simulink model "slam_check"  (R2013b)
settings: Solver=ode3  StartTime=0.0  StopTime=3  FixedStep=0.1  RelTol=1e-3
undefined symbols (not defined in the file): DiscIntNeverNeededParam
settings Model: Creator=chida  LastModifiedBy=chida
settings DataIOCC: SignalLoggingSaveFormat=ModelDataLogs
settings DebuggingCC: MultiTaskDSMMsg=warning  MultiTaskCondExecSysMsg=none
settings RTWCC: IncludeERTFirstTime=on

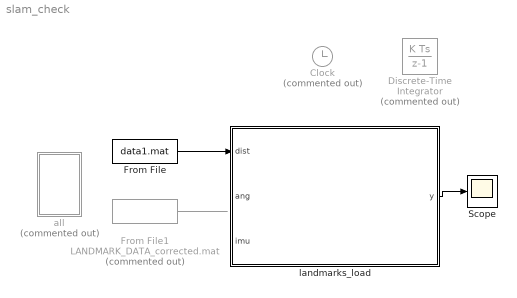
== system slam_check ==
  Clock : Clock  Commented=on
  Discrete-Time Integrator : DiscreteIntegrator  Commented=on  ICPrevOutput=DiscIntNeverNeededParam  ICPrevScaledInput=DiscIntNeverNeededParam
  From File : FromFile  FileName=data1.mat  SampleTime=0
  From File1 : FromFile  Commented=on  FileName=LANDMARK_DATA_corrected.mat  SampleTime=0
  Scope : Scope
  all : Subsystem  Commented=on
  landmarks_load : MATLAB Function  TreatAsAtomicUnit=on
  wires:
  From File/1 -> landmarks_load/1(dist)
  landmarks_load/1(y) -> Scope/1
  From File1/1 -> ?

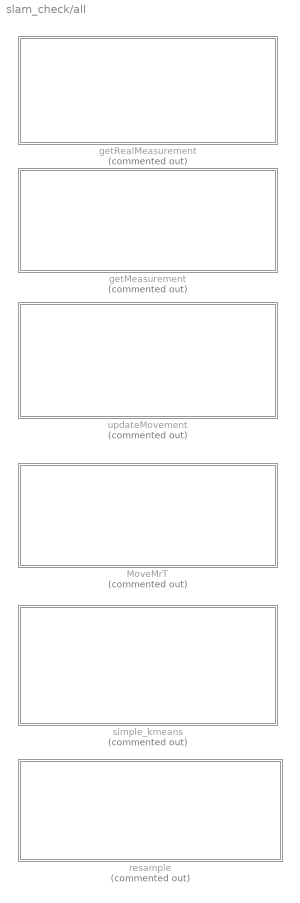
== system slam_check/all ==
  MoveMrT : MATLAB Function  Commented=on  TreatAsAtomicUnit=on
  getMeasurement : MATLAB Function  Commented=on  TreatAsAtomicUnit=on
  getRealMeasurement : MATLAB Function  Commented=on  TreatAsAtomicUnit=on
  resample : MATLAB Function  Commented=on  TreatAsAtomicUnit=on
  simple_kmeans : MATLAB Function  Commented=on  TreatAsAtomicUnit=on
  updateMovement : MATLAB Function  Commented=on  TreatAsAtomicUnit=on

== matlab function slam_check/all/getMeasurement ==
%%%%%%%%%%%%%%%%%%%%%%%%%%%%%%%%%%%%%%%%%%%%%%%%%%%%%%%%%%%%%%%%%%%%%%
%  Copyright 2010 Randolph Voorhies
%  This program is free software: you can redistribute it and/or modify
%  it under the terms of the GNU General Public License as published by
%  the Free Software Foundation, either version 3 of the License, or
%  (at your option) any later version.
%
%  This program is distributed in the hope that it will be useful,
%  but WITHOUT ANY WARRANTY; without even the implied warranty of
%  MERCHANTABILITY or FITNESS FOR A PARTICULAR PURPOSE.  See the
%  GNU General Public License for more details.
%
%  You should have received a copy of the GNU General Public License
%  along with this program.  If not, see <http://www.gnu.org/licenses/>.
%%%%%%%%%%%%%%%%%%%%%%%%%%%%%%%%%%%%%%%%%%%%%%%%%%%%%%%%%%%%%%%%%%%%%%   
% function [z, H] = getMeasurement(pos, landmark_pos, observation_variance)
function getMeasurement
%   Given a landmark position and a robot position, this method will return a
%   "measurement" z that contains the distance and the angle to the landmark.
%   Gaussian random noise is added to both based on the variances given in the
%   diagonal of the observation_variance matrix. Note that this method is used
%   both to take a "real" measurement in the simulation, as well as to assess 
%   what kind of measurement each of our hypothetical particles would take.
%   This method also computes the Jacobian of the measurent function for use
%   in an extended Kalman filter.

    pos=[0.173668180001441;1.04972580955013;0.201278478584753];
    landmark_pos=[0.167872078898977,3.28720981409093];
    observation_variance=[0 0];


  % Compute the distance from the current position to the landmark, and add
  % some Gaussian noise to make things interesting. Note that we are using
  % a smaller variance in this Gaussian distribution, as the algorithm seems
  % to work better when it underestimates the quality of the sensor. 
  vector_to_landmark = [landmark_pos(1) - pos(1); landmark_pos(2) - pos(2)];
  landmark_distance = norm(vector_to_landmark);
%   landmark_distance = landmark_distance + normrnd(0, observation_variance(1)*.25);
  landmark_distance = landmark_distance;


  % Compute the angle from the given pos to the landmark
  landmark_angle = atan2(vector_to_landmark(1), vector_to_landmark(2))-pos(3);
%   landmark_angle = landmark_angle + normrnd(0, observation_variance(2)*.25);
landmark_angle = landmark_angle;

  % Compute the Jacobian of this measurement function
  q = landmark_distance^2.0;
%   H = [-(landmark_pos(1) - pos(1))/sqrt(q), -(landmark_pos(2) - pos(2))/sqrt(q), 0.0;
%         (landmark_pos(2) - pos(2))/q,       -(landmark_pos(1) - pos(1))/q,      -1.0;
%         0.0,                                0.0,                               1.0];

  H = [-(landmark_pos(1) - pos(1))/landmark_distance, -(landmark_pos(2) - pos(2))/landmark_distance;
        (landmark_pos(2) - pos(2))/q,       -(landmark_pos(1) - pos(1))/q];




  z = [landmark_distance; 
       landmark_angle];
       %0]; remove signifier (not using color data)
end

== matlab function slam_check/all/getRealMeasurement ==
%%%%%%%%%%%%%%%%%%%%%%%%%%%%%%%%%%%%%%%%%%%%%%%%%%%%%%%%%%%%%%%%%%%%%%
%  Copyright 2010 Randolph Voorhies
%  This program is free software: you can redistribute it and/or modify
%  it under the terms of the GNU General Public License as published by
%  the Free Software Foundation, either version 3 of the License, or
%  (at your option) any later version.
%
%  This program is distributed in the hope that it will be useful,
%  but WITHOUT ANY WARRANTY; without even the implied warranty of
%  MERCHANTABILITY or FITNESS FOR A PARTICULAR PURPOSE.  See the
%  GNU General Public License for more details.
%
%  You should have received a copy of the GNU General Public License
%  along with this program.  If not, see <http://www.gnu.org/licenses/>.
%%%%%%%%%%%%%%%%%%%%%%%%%%%%%%%%%%%%%%%%%%%%%%%%%%%%%%%%%%%%%%%%%%%%%%   
% function [z, H] = getRealMeasurement(pos, landmark_pos, observation_variance)
function getRealMeasurement
%   Given a landmark position and a robot position, this method will return a
%   "measurement" z that contains the distance and the angle to the landmark.
%   Gaussian random noise is added to both based on the variances given in the
%   diagonal of the observation_variance matrix. Note that this method is used
%   both to take a "real" measurement in the simulation, as well as to assess 
%   what kind of measurement each of our hypothetical particles would take.
%   This method also computes the Jacobian of the measurent function for use
%   in an extended Kalman filter.

    pos=[0.173668180001441;1.04972580955013;0.201278478584753];
    landmark_pos=[0.167872078898977,3.28720981409093];
    observation_variance=[0 0];

  % Compute the distance from the current position to the landmark, and add
  % some Gaussian noise to make things interesting. Note that we are using
  % a smaller variance in this Gaussian distribution, as the algorithm seems
  % to work better when it underestimates the quality of the sensor. 
%   vector_to_landmark = [landmark_pos(1) - pos(1); landmark_pos(2) - pos(2)];
%   landmark_distance = norm(vector_to_landmark);
%   landmark_distance = landmark_distance + normrnd(0, observation_variance(1)*.25);

%   % Compute the angle from the given pos to the landmark
%   landmark_angle = atan2(vector_to_landmark(2), vector_to_landmark(1));
%   landmark_angle = landmark_angle + normrnd(0, observation_variance(2)*.25);

  landmark_angle=landmark_pos(1);
  landmark_distance=landmark_pos(2);

  % Compute the Jacobian of this measurement function
  q = landmark_distance^2.0;
%   H = [-(landmark_pos(1) - pos(1))/sqrt(q), -(landmark_pos(2) - pos(2))/sqrt(q), 0.0;
%         (landmark_pos(2) - pos(2))/q,       -(landmark_pos(1) - pos(1))/q,      -1.0;
%         0.0,                                0.0,                               1.0];
    
    H = [-(landmark_pos(1) - pos(1))/sqrt(q), -(landmark_pos(2) - pos(2))/sqrt(q);
        (landmark_pos(2) - pos(2))/q,       -(landmark_pos(1) - pos(1))/q];


  z = [landmark_distance; 
       landmark_angle];
       %0]; not using color ID
end

== matlab function slam_check/all/updateMovement ==
%%%%%%%%%%%%%%%%%%%%%%%%%%%%%%%%%%%%%%%%%%%%%%%%%%%%%%%%%%%%%%%%%%%%%%
%  Copyright 2010 Randolph Voorhies
%  This program is free software: you can redistribute it and/or modify
%  it under the terms of the GNU General Public License as published by
%  the Free Software Foundation, either version 3 of the License, or
%  (at your option) any later version.
%
%  This program is distributed in the hope that it will be useful,
%  but WITHOUT ANY WARRANTY; without even the implied warranty of
%  MERCHANTABILITY or FITNESS FOR A PARTICULAR PURPOSE.  See the
%  GNU General Public License for more details.
%
%  You should have received a copy of the GNU General Public License
%  along with this program.  If not, see <http://www.gnu.org/licenses/>.
%%%%%%%%%%%%%%%%%%%%%%%%%%%%%%%%%%%%%%%%%%%%%%%%%%%%%%%%%%%%%%%%%%%%%%   
% function newpos = updateMovement(pos, movement, variance)
function updateMovement
% Compute how the robot should move from "pos" given the requested movement and
% some Gaussian random noise using a very simple motion model. This method is
% used to move the simulated robot as well as each of the hypothetical
% particles.

   pos=[0.173668180001441;1.04972580955013;0.201278478584753];
movement=[0.6000 0.6000];
variance=[0.100000000000000;0.100000000000000];
   

  % Add some Gaussian random noise to the movement. Note that we are using
  % a smaller variance in this Gaussian distribution, as the algorithm seems
  % to work better when it underestimates the quality of the robot plant. 
  speed    = normrnd(movement(1), variance(1)*.25);
  rotation = normrnd(movement(2), variance(2)*.25);

  delta = zeros(3,1);
  delta(1,1) = cos(pos(3)+rotation)*speed;
  delta(2,1) = sin(pos(3)+rotation)*speed;
  delta(3,1) = rotation;

  newpos = pos+delta;
end

== matlab function slam_check/all/MoveMrT ==
%%%%%%%%%%%%%%%%%%%%%%%%%%%%%%%%%%%%%%%%%%%%%%%%%%%%%%%%%%%%%%%%%%%%%%
%  Nick DiLeo 2014
%  Villanova University

%%%%%%%%%%%%%%%%%%%%%%%%%%%%%%%%%%%%%%%%%%%%%%%%%%%%%%%%%%%%%%%%%%%%%%   
% function newpos = MoveMrT(pos, movement, variance,dt)
function MoveMrT
% Compute how the MrT robot should move from "pos" given the requested movement and
% some Gaussian random noise using a very simple motion model. This method is
% used to move the each of the particles.
pos=[0.173668180001441;1.04972580955013;0.201278478584753];
movement=[0.6000 0.6000];
variance=[0.100000000000000;0.100000000000000];
dt=0.3652;

  % Add some Gaussian random noise to the movement. Note that we are using
  % a smaller variance in this Gaussian distribution, as the algorithm seems
  % to work better when it underestimates the quality of the robot plant. 
  l_wheel_des    = normrnd(movement(1), variance(1));
  r_wheel_des = normrnd(movement(2), variance(2));
  wheel_radius = 0.04445; %m 
%  wheel_radius = 0.06; %m 
  wheel_base = 0.3175; %m
  
  %wheel velocities
  vel_right = r_wheel_des*wheel_radius;
  vel_left = l_wheel_des*wheel_radius;
  
  v_robot = (vel_right+vel_left)/2; %forward velocity of robot m/s
  omega_robot = (vel_left-vel_right)/wheel_base; %angular velocity of robot
  
  x_dot = sin(pos(3))*v_robot;
  y_dot = cos(pos(3))*v_robot;
    
  delta = zeros(3,1);
  delta(1,1) = x_dot*dt;
  delta(2,1) = y_dot*dt;
  delta(3,1) = omega_robot*dt;
  newpos = pos+delta;
end

== matlab function slam_check/all/resample ==
%%%%%%%%%%%%%%%%%%%%%%%%%%%%%%%%%%%%%%%%%%%%%%%%%%%%%%%%%%%%%%%%%%%%%%
%  Copyright 2010 Randolph Voorhies
%  This program is free software: you can redistribute it and/or modify
%  it under the terms of the GNU General Public License as published by
%  the Free Software Foundation, either version 3 of the License, or
%  (at your option) any later version.
%
%  This program is distributed in the hope that it will be useful,
%  but WITHOUT ANY WARRANTY; without even the implied warranty of
%  MERCHANTABILITY or FITNESS FOR A PARTICULAR PURPOSE.  See the
%  GNU General Public License for more details.
%
%  You should have received a copy of the GNU General Public License
%  along with this program.  If not, see <http://www.gnu.org/licenses/>.
%%%%%%%%%%%%%%%%%%%%%%%%%%%%%%%%%%%%%%%%%%%%%%%%%%%%%%%%%%%%%%%%%%%%%%   
% function newParticles  = resample(oldParticles)
function resample
% Resample a group of particles such that those with higher weights have a
% higher chance of being replicated, and those with low weights have a high
% chance of disappearing
%% for oldparticles
 num_particles=50;
 field1='w';            value1=1.0/num_particles;
 field2='position';       value2=[0;0;0];
 field3='num_landmarks';       value3=0;
 field4='lm_weight';       value4=1.0/num_particles;
 
 part = struct(field1,value1,field2,value2,field3,value3,field4,value4);
 oldParticles=repmat(part,num_particles);
 
 xsiva=0;
 ysiva=0;
 rotsiva=0;
 
 for siva=1:num_particles
     oldParticles(siva).w=rand(1,1);
 end
 
 %% repeat for new particles
 
 newParticles=repmat(part,num_particles);
 

%% Actual
  weightSum = 0;
  for i=1:length(oldParticles)
    weightSum = weightSum + oldParticles(i).w;
  end
  
  for i=1:length(oldParticles)
    oldParticles(i).w = oldParticles(i).w/weightSum;
  end

  M = length(oldParticles);

%   newParticles = [];

  r = rand / M;

  c = oldParticles(1).w;

  i = 1;

  l=1;
  for m=1:M
    U = r + (m-1) * M^(-1);

    while U > c
      i = i+1;
      c = c+oldParticles(i).w;
    end
    newParticles(l) = oldParticles(i);
    l=l+1;
  end

  for i=1:length(newParticles)
    newParticles(i).w = 1.0/length(newParticles);
  end

end

== matlab function slam_check/all/simple_kmeans ==
function simple_kmeans


K = 4;
dim = 3;
variance = 1;
sdev = sqrt(variance);

cluster1 = sdev*randn(200,dim) + kron(ones(200,1),[0,0,0]);
cluster2 = sdev*randn(300,dim) + kron(ones(300,1),[0,0,6]);
cluster3 = sdev*randn(100,dim) + kron(ones(100,1),[0,6,0]);
cluster4 = sdev*randn(500,dim) + kron(ones(500,1),[6,0,0]);

% Build data matrix
X = [cluster1 ; cluster2 ; cluster3; cluster4];

maxerr = 0;


[Ndata, dims] = size(X);
dist = zeros(1,K);
means=[0.5 0.5 0.5;0.5 0.5 0.5;0.5 0.5 0.5;0.5 0.5 0.5];
coder.varsize('means', [6 6]);
% means[1100][3];
% means = double.empty(1100,3);
% means= zeros(1100,3);
% Initial prototype assignment (arbitrary)
for i=1:K-1
   means(i,:) = X(i,:);
end
means(K,:) = mean(X(K:Ndata,:));

cmp = 1 + maxerr;
while (cmp > maxerr)
   % Sums (class) and data counters (Nclass) initialization
   class = zeros(K,dims);
   Nclass = zeros(K,1);

   % Groups each elements to the nearest prototype
   for i=1:Ndata
      for j=1:K
         % Euclidean distance from data to each prototype
         dist(j) = norm(X(i,:)-means(j,:))^2;
      end
      % Find indices of minimum distance
      index_min = find(~(dist-min(dist)));
      % If there are multiple min distances, decide randomly
      index_min = index_min(ceil(length(index_min)*rand));
      class(index_min,:) = class(index_min,:) + X(i,:);
      Nclass(index_min) = Nclass(index_min) + 1;
   end
   for i=1:K
      class(i,:) = class(i,:) / Nclass(i);
   end

   % Compare results with previous iteration
   cmp = 0;
   for i=1:K
      cmp = norm(class(i,:)-means(i,:)); 
   end

   % Prototype update
   means = class;
end

% Nmeans = Nclass;

== matlab function slam_check/landmarks_load ==
  data: y output; dist input; ang input; imu input
function y  = landmarks_load(dist,ang,imu)
%%[time, dtime, r_wheel desired speed, r_wheel measured speed, 
%l_wheel desired speed, l_wheel measured speed];

%% Init block run this block only once.

persistent timestep particles; 
timestep=2;
num_particles = 50;
% % The maximum distance from which our sensor can sense a landmark
max_read_distance = 5;
min_read_distance = 0.3;
min_read_angle = -22*pi/180; %radians- maximum read angle
max_read_angle = 22*pi/180;
% The initial starting position of the robot
avg_robot_position = [0;      % x %Use UTM coordinates from GPS 
                 0;     % y
                 0];  % rotation               
% The Gaussian variance of the movement commands
movement_variance = [.1;   % Left wheel
                     .1]; % Right_wheel
M = [movement_variance(1), 0.0;
     0.0, movement_variance(2)];
measurement_variance = [0.01;    % Distance
                        0.01];   % Angle
R = [measurement_variance(1), 0.0;
     0.0, measurement_variance(2)];
 default_importance=0.0000001; 
 pos_history = [];
 
 if ~isempty(particles)
    % Create the particles and initialize them all to be in the same initial
    % position.
    %  field1='w';            value1=1.0/num_particles;
    %  field2='position';       value2=avg_robot_position;
    %  field3='num_landmarks';       value3=0;
    %  field4='lm_weight';       value4=1.0/num_particles;
    %  part = struct(field1,value1,field2,value2,field3,value3,field4,value4);
    %  particles=repmat(part,50);
    particles=repmat(struct('w',1.0/num_particles,'position',avg_robot_position,'num_landmarks',zeros(1,300),'lm_weight',repmat(1.0/num_particles,2,15),'landmarks',repmat(struct('pos',zeros(1,2),'E',zeros(6,6),'counter',0,'size_E',zeros(1,2)),1,15)),1,50);
    avg_robot_position = average_pos(particles,num_particles);
 end
 
 
 

%% Load data
landmark1 = [dist(1),ang(1)];
landmark2 = [dist(2),ang(2)];
landmark3 = [dist(3),ang(3)];
landmark4 = [dist(4),ang(4)];
landmark5 = [dist(5),ang(5)];
landmark6 = [dist(6),ang(6)];
landmark7 = [dist(7),ang(7)];
landmark8 = [dist(8),ang(8)];
landmark9 = [dist(9),ang(9)];
landmark10 = [dist(10),ang(10)];
landmark11 = [dist(11),ang(11)];
landmark12 = [dist(12),ang(12)];

roll=imu(1);
pitch=imu(2);
yaw=imu(3);

dt=0;
r_wheel_des= 0;
r_wheel_mes= 0;
l_wheel_des= 0;
l_wheel_mes= 0;


  %% Move the actual particles
  % Needs replaced for new model.
  
  
  for pIdx = 1:num_particles
      
      %particles(pIdx).position = MoveMrT(particles(pIdx).position, [data(timestep,3) data(timestep,5)],movement_variance,data(timestep,2));
      %newpos = MoveMrT(pos, movement, variance,dt
    l_wheel_des    = normrnd(l_wheel_des, movement_variance(1));
    r_wheel_des = normrnd(r_wheel_des, movement_variance(2));
    wheel_radius = 0.04445; %m 
    wheel_base = 0.3175; %m
  
  %wheel velocities
    vel_right = r_wheel_des*wheel_radius;
    vel_left = l_wheel_des*wheel_radius;
  
    v_robot = (vel_right+vel_left)/2; %forward velocity of robot m/s
    omega_robot = (vel_left-vel_right)/wheel_base; %angular velocity of robot
  
    x_dot = sin(particles(pIdx).position(3))*v_robot;
    y_dot = cos(particles(pIdx).position(3))*v_robot;
    
    particles(pIdx).position(1) = particles(pIdx).position(1)+x_dot*dt;
    particles(pIdx).position(2) =  particles(pIdx).position(2)+y_dot*dt;
    particles(pIdx).position(3) = particles(pIdx).position(3)+omega_robot*dt;
      
  end
  
  
  z_real=[0;0];
  %%
  % Try to take a reading from each landmark
  doResample = false;
% The input got from landmarks
  collected_data=[-0.119955307371067,2.31463298709723,0.270433587697713,2.06920493403612,0.270712733973202,2.06936515522061,-0.119955307371067,2.31463298709723,0.270433587697713,2.06920493403612,0.270712733973202,2.06936515522061];
  [,cols,]=find(collected_data ~= 0);
  if (isempty(cols)==0)% if the cols is not empty
      doResample=true; %if there is new measurement, then resample particles
  end
  

  if (doResample==true)
      [r,c]=size(cols);
      shiva=1;
      for lIdx = 1:2:c %amount of visible landmarks
        real_landmark = [collected_data(1,lIdx),collected_data(1,lIdx+1)];
        % Take a real (noisy) measurement from the robot to the landmark
%         [z_real(:,lIdx), G(:,:,lIdx)] = getRealMeasurement(avg_robot_position, real_landmark, [0 0]);
%         function [z, H] = getRealMeasurement(pos, landmark_pos, observation_variance)
        
        landmark_angle=real_landmark(1);
        landmark_distance=real_landmark(2);

        % Compute the Jacobian of this measurement function
        q = landmark_distance^2.0;
    
        H = [-(real_landmark(1) - avg_robot_position(1))/sqrt(q), -(real_landmark(2) - avg_robot_position(2))/sqrt(q);
        (real_landmark(2) - avg_robot_position(2))/q,       -(real_landmark(1) - avg_robot_position(1))/q];


        z_real = [landmark_distance; landmark_angle];
%         read_distance(shiva) = landmark_distance;
%         read_angle(shiva)    = landmark_angle;
      end
      
      
      
      %% Actual for each particle calculation.
      
      
      for pIdx = 1:num_particles               
%           
% %           particles(pIdx).lm_weight=[];
% %           clear z_p H Q
          for j=1:particles(pIdx).num_landmarks(timestep-1)
%                 
% %               [z_p(:,j), H(:,:,j)] = getMeasurement(particles(pIdx).position, particles(pIdx).landmarks(j).pos, [0 0]);
% %               function [z, H] = getMeasurement(pos, landmark_pos, observation_variance)
                observation_variance=[0 0];
                vector_to_landmark = [particles(pIdx).landmarks(j).pos(1) - particles(pIdx).position(1); particles(pIdx).landmarks(j).pos(2) - particles(pIdx).position(2)];
                landmark_distance = norm(vector_to_landmark);
                %   landmark_distance = landmark_distance + normrnd(0, observation_variance(1)*.25);
                landmark_distance = landmark_distance;

                 % Compute the angle from the given pos to the landmark
                landmark_angle = atan2(vector_to_landmark(1), vector_to_landmark(2))-particles(pIdx).position(3);
                %   landmark_angle = landmark_angle + normrnd(0, observation_variance(2)*.25);
                landmark_angle = landmark_angle;

                  % Compute the Jacobian of this measurement function
                q = landmark_distance^2.0;
                %   H = [-(landmark_pos(1) - pos(1))/sqrt(q), -(landmark_pos(2) - pos(2))/sqrt(q), 0.0;
                %         (landmark_pos(2) - pos(2))/q,       -(landmark_pos(1) - pos(1))/q,      -1.0;
                %         0.0,                                0.0,                               1.0];

                H = [-(particles(pIdx).landmarks(j).pos(1) - particles(pIdx).position(1))/landmark_distance, -(particles(pIdx).landmarks(j).pos(2) - particles(pIdx).position(2))/landmark_distance;
                        (particles(pIdx).landmarks(j).pos(2) - particles(pIdx).position(2))/q,       -(particles(pIdx).landmarks(j).pos(1) - particles(pIdx).position(1))/q];
 
                z_p = [landmark_distance; 
                    landmark_angle];
% 
              for measured_lm=1:size(z_real,2) 
                residual = z_real(:,measured_lm) - z_p(:,j);
                Q=zeros(size(R));
                E=zeros(particles(pIdx).landmarks(j).size_E);
                E=particles(pIdx).landmarks(j).E(1:particles(pIdx).landmarks(j).size_E(1,1),1:particles(pIdx).landmarks(j).size_E(1,2));
%                 E=particles(pIdx).landmarks(j).E()

                Q(:,:,j) = H(:,:,j)' * E * H(:,:,j) + R;             
                particles(pIdx).lm_weight(measured_lm,j) = particles(pIdx).w * norm(2*pi*Q(:,:,j)).^(-1/2)*exp(-1/2*(residual)'*inv(Q(:,:,j))*(residual));
              end
          end
          
                    %probably going to delete this hold on for now
          %           particles(pIdx).lm_weight(particles(pIdx).num_landmarks(timestep-1)+1) = 0.09; %importance factor, new feature
          particles(pIdx).num_landmarks(timestep)=particles(pIdx).num_landmarks(timestep-1);
          %           clear c_hat
          
          cost_table=zeros(size(z_real,2),particles(pIdx).num_landmarks(timestep-1));
          cost_table(1:size(z_real,2),1:particles(pIdx).num_landmarks(timestep-1))=particles(pIdx).lm_weight(1:particles(pIdx).num_landmarks(timestep-1));
% need to work on this          cost_table(1:size(z_real,2),particles(pIdx).num_landmarks(timestep-1)+1:particles(pIdx).num_landmarks(timestep-1)+size(z_real,2))=default_importance*eye(size(z_real,2));
          if(isempty(max(max(cost_table)))) particles(pIdx).w=0;
%           else particles(pIdx).w=max(max(cost_table));
          end
          [~, idx_hold]=max(cost_table,[],1); %this is the max correseponding for each measurement
          for i=1:size(cost_table,2)
             idx_zero=setdiff([1:size(cost_table,1)],idx_hold(i));
             cost_table(idx_zero,i)=0;
          end

          
          
          
          
          
          
          
          
      end % End of pIdx = 1:num_particles
      
      
      
      
      
      
      
      
      
      
      
      
      
      
      
      
      
      
      
      
      
      
      
      
      
%% the end for the condition to make sure if there is no measurements to not alculate things.      
  end
  
  
  
  
  
  
  
  
  
  
  
  
  
  
        
     




y= r_wheel_des;


end


function avg_robot_position = average_pos(particles,num_particles)
 xsiva=0;
 ysiva=0;
 rotsiva=0;
 
 for siva=1:num_particles
     xsiva=xsiva+particles(siva).position(1);
     ysiva=ysiva+particles(siva).position(2);
     rotsiva=rotsiva+particles(siva).position(3);
 end

avg_robot_position = [xsiva/num_particles; ysiva/num_particles; rotsiva/num_particles];

end
